simulink subsystem "PvtSubSys_VIE"  (R2020b)
settings: Solver=VariableStepAuto  StartTime=0.0  StopTime=10.0  RelTol=1e-3
undefined symbols (not defined in the file): P_Global_CharSpd_ms, P_Global_FrontAxleToCenter_m, P_Global_RearAxleToCenter_m, P_Global_SideSlipAnglefactor, P_Global_SteeringAngleRatio, P_Global_WheelBase_m, P_Global_WheelTrack_m
libraries: simulink x16
(part 1 of 2)
settings Model: Creator=GW00184765  LastModifiedBy=GW00201118

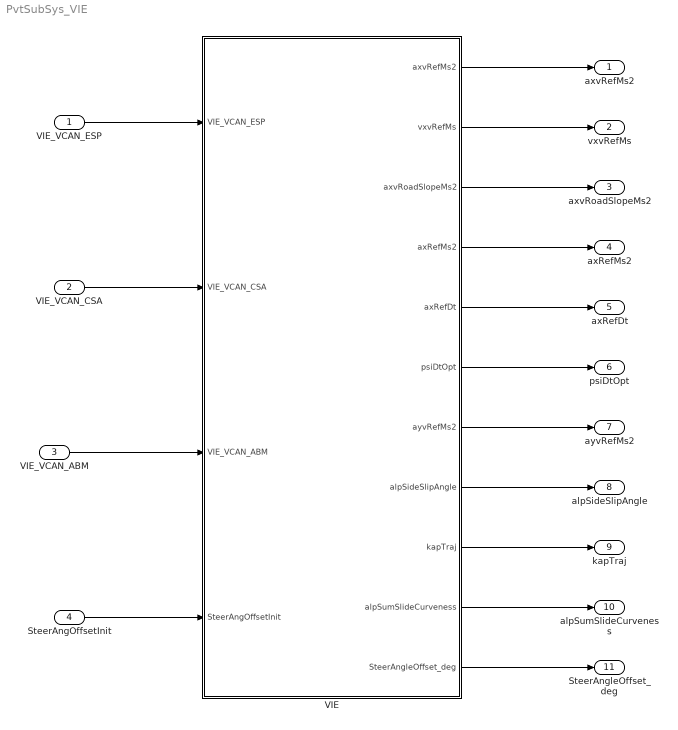
== system PvtSubSys_VIE ==
  VIE_VCAN_ESP : Inport  OutDataTypeStr=Bus: VCAN_ESP_MSG_BUS  PortDimensions=1  BusOutputAsStruct=on
  VIE_VCAN_CSA : Inport  Port=2  OutDataTypeStr=Bus: VCAN_CSA_MSG_BUS  PortDimensions=1  BusOutputAsStruct=on
  VIE_VCAN_ABM : Inport  Port=3  OutDataTypeStr=Bus: VCAN_ABM_MSG_BUS  PortDimensions=1  BusOutputAsStruct=on
  SteerAngOffsetInit : Inport  Port=4
  VIE : Subsystem
  axvRefMs2 : Outport  OutDataTypeStr=single  PortDimensions=1  BusOutputAsStruct=on
  vxvRefMs : Outport  Port=2  OutDataTypeStr=single  PortDimensions=1  BusOutputAsStruct=on
  axvRoadSlopeMs2 : Outport  Port=3  OutDataTypeStr=single  PortDimensions=1  BusOutputAsStruct=on
  axRefMs2 : Outport  Port=4  OutDataTypeStr=single  PortDimensions=1  BusOutputAsStruct=on
  axRefDt : Outport  Port=5  OutDataTypeStr=single  PortDimensions=1  BusOutputAsStruct=on
  psiDtOpt : Outport  Port=6  OutDataTypeStr=single  PortDimensions=1  BusOutputAsStruct=on
  ayvRefMs2 : Outport  Port=7  OutDataTypeStr=single  PortDimensions=1  BusOutputAsStruct=on
  alpSideSlipAngle : Outport  Port=8  OutDataTypeStr=single  PortDimensions=1  BusOutputAsStruct=on
  kapTraj : Outport  Port=9  OutDataTypeStr=single  PortDimensions=1  BusOutputAsStruct=on
  alpSumSlideCurveness : Outport  Port=10  OutDataTypeStr=single  PortDimensions=1  BusOutputAsStruct=on
  SteerAngleOffset_deg : Outport  Port=11  OutDataTypeStr=single  PortDimensions=1  BusOutputAsStruct=on
  wires:
  VIE_VCAN_ABM/1 -> VIE/3(VIE_VCAN_ABM)
  VIE_VCAN_CSA/1 -> VIE/2(VIE_VCAN_CSA)
  VIE_VCAN_ESP/1 -> VIE/1(VIE_VCAN_ESP)
  VIE/9(kapTraj) -> kapTraj/1
  VIE/11(SteerAngleOffset_deg) -> SteerAngleOffset_deg/1
  VIE/8(alpSideSlipAngle) -> alpSideSlipAngle/1
  VIE/7(ayvRefMs2) -> ayvRefMs2/1
  VIE/2(vxvRefMs) -> vxvRefMs/1
  VIE/5(axRefDt) -> axRefDt/1
  VIE/4(axRefMs2) -> axRefMs2/1
  VIE/10(alpSumSlideCurveness) -> alpSumSlideCurveness/1
  VIE/3(axvRoadSlopeMs2) -> axvRoadSlopeMs2/1
  VIE/1(axvRefMs2) -> axvRefMs2/1
  VIE/6(psiDtOpt) -> psiDtOpt/1
  SteerAngOffsetInit/1 -> VIE/4(SteerAngOffsetInit)

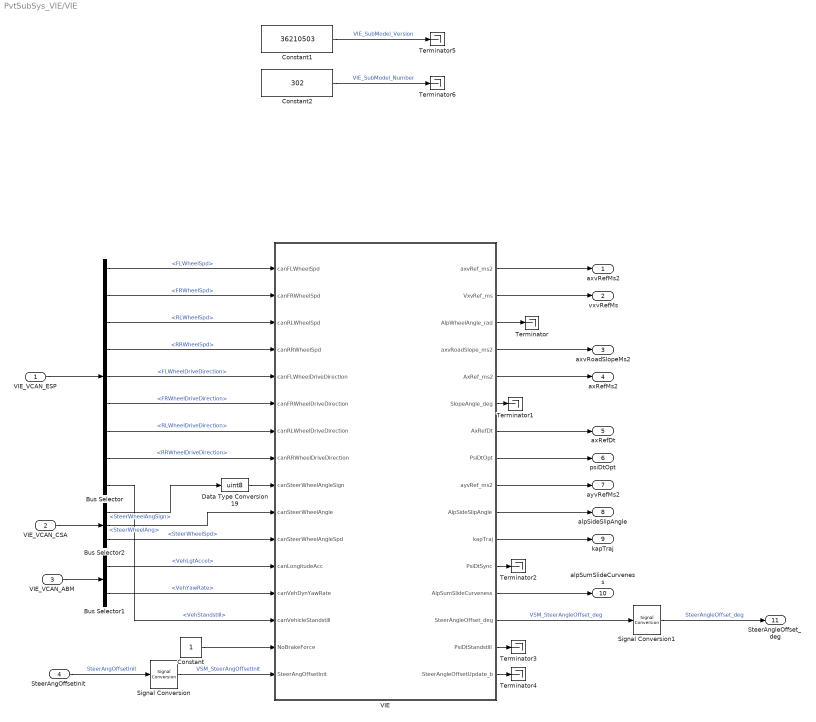
== system PvtSubSys_VIE/VIE ==
  VIE_VCAN_ESP : Inport  OutDataTypeStr=Bus: VCAN_ESP_MSG_BUS  PortDimensions=1  BusOutputAsStruct=on
  VIE_VCAN_CSA : Inport  Port=2  OutDataTypeStr=Bus: VCAN_CSA_MSG_BUS  PortDimensions=1  BusOutputAsStruct=on
  VIE_VCAN_ABM : Inport  Port=3  OutDataTypeStr=Bus: VCAN_ABM_MSG_BUS  PortDimensions=1  BusOutputAsStruct=on
  SteerAngOffsetInit : Inport  Port=4
  Bus Selector : BusSelector  OutputSignals=FLWheelSpd,FRWheelSpd,RLWheelSpd,RRWheelSpd,FLWheelDriveDirection,FRWheelDriveDirection,RLWheelDriveDirection,RRWheelDriveDirection,VehStandstill
  Bus Selector1 : BusSelector  OutputSignals=VehLgtAccel,VehYawRate
  Bus Selector2 : BusSelector  OutputSignals=SteerWheelAngSign,SteerWheelAng,SteerWheelSpd
  Constant : Constant  OutDataTypeStr=single
  Constant1 : Constant  Value=36210503  OutDataTypeStr=uint32
  Constant2 : Constant  Value=302  OutDataTypeStr=uint32
  Data Type Conversion19 : DataTypeConversion  OutDataTypeStr=uint8
  Signal Conversion : SignalConversion  OverrideOpt=off
  Signal Conversion1 : SignalConversion  OverrideOpt=off
  Terminator{,1..6} (7 alike) : Terminator
  VIE : Subsystem
  axvRefMs2 : Outport  OutDataTypeStr=single  PortDimensions=1  BusOutputAsStruct=on
  vxvRefMs : Outport  Port=2  OutDataTypeStr=single  PortDimensions=1  BusOutputAsStruct=on
  axvRoadSlopeMs2 : Outport  Port=3  OutDataTypeStr=single  PortDimensions=1  BusOutputAsStruct=on
  axRefMs2 : Outport  Port=4  OutDataTypeStr=single  PortDimensions=1  BusOutputAsStruct=on
  axRefDt : Outport  Port=5  OutDataTypeStr=single  PortDimensions=1  BusOutputAsStruct=on
  psiDtOpt : Outport  Port=6  OutDataTypeStr=single  PortDimensions=1  BusOutputAsStruct=on
  ayvRefMs2 : Outport  Port=7  OutDataTypeStr=single  PortDimensions=1  BusOutputAsStruct=on
  alpSideSlipAngle : Outport  Port=8  OutDataTypeStr=single  PortDimensions=1  BusOutputAsStruct=on
  kapTraj : Outport  Port=9  OutDataTypeStr=single  PortDimensions=1  BusOutputAsStruct=on
  alpSumSlideCurveness : Outport  Port=10  OutDataTypeStr=single  PortDimensions=1  BusOutputAsStruct=on
  SteerAngleOffset_deg : Outport  Port=11  OutDataTypeStr=single  PortDimensions=1  BusOutputAsStruct=on
  wires:
  VIE/14(SteerAngleOffset_deg) -> Signal Conversion1/1  "VSM_SteerAngleOffset_deg"
  Signal Conversion/1 -> VIE/16(SteerAngOffsetInit)  "VSM_SteerAngOffsetInit"
  Constant1/1 -> Terminator5/1  "VIE_SubModel_Version"
  Constant2/1 -> Terminator6/1  "VIE_SubModel_Number"
  SteerAngOffsetInit/1 -> Signal Conversion/1  "SteerAngOffsetInit"
  VIE/15(PsiDtStandstill) -> Terminator3/1
  VIE/3(AlpWheelAngle_rad) -> Terminator/1
  Signal Conversion1/1 -> SteerAngleOffset_deg/1  "SteerAngleOffset_deg"
  VIE/13(AlpSumSlideCurveness) -> alpSumSlideCurveness/1
  Data Type Conversion19/1 -> VIE/9(canSteerWheelAngleSign)
  VIE/4(axvRoadSlope_ms2) -> axvRoadSlopeMs2/1
  VIE/6(SlopeAngle_deg) -> Terminator1/1
  VIE/10(AlpSideSlipAngle) -> alpSideSlipAngle/1
  VIE/5(AxRef_ms2) -> axRefMs2/1
  VIE/11(kapTraj) -> kapTraj/1
  VIE/7(AxRefDt) -> axRefDt/1
  VIE/8(PsiDtOpt) -> psiDtOpt/1
  Bus Selector/7 -> VIE/7(canRLWheelDriveDirection)  "<RLWheelDriveDirection>"
  Bus Selector/6 -> VIE/6(canFRWheelDriveDirection)  "<FRWheelDriveDirection>"
  VIE_VCAN_ABM/1 -> Bus Selector1/1
  Constant/1 -> VIE/15(NoBrakeForce)
  Bus Selector/8 -> VIE/8(canRRWheelDriveDirection)  "<RRWheelDriveDirection>"
  VIE/12(PsiDtSync) -> Terminator2/1
  Bus Selector1/2 -> VIE/13(canVehDynYawRate)  "<VehYawRate>"
  Bus Selector2/3 -> VIE/11(canSteerWheelAngleSpd)  "<SteerWheelSpd>"
  Bus Selector2/1 -> Data Type Conversion19/1  "<SteerWheelAngSign>"
  VIE/9(ayvRef_ms2) -> ayvRefMs2/1
  Bus Selector/9 -> VIE/14(canVehicleStandstill)  "<VehStandstill>"
  Bus Selector2/2 -> VIE/10(canSteerWheelAngle)  "<SteerWheelAng>"
  Bus Selector/5 -> VIE/5(canFLWheelDriveDirection)  "<FLWheelDriveDirection>"
  VIE_VCAN_CSA/1 -> Bus Selector2/1
  Bus Selector/3 -> VIE/3(canRLWheelSpd)  "<RLWheelSpd>"
  VIE/2(VxvRef_ms) -> vxvRefMs/1
  Bus Selector1/1 -> VIE/12(canLongitudeAcc)  "<VehLgtAccel>"
  Bus Selector/1 -> VIE/1(canFLWheelSpd)  "<FLWheelSpd>"
  VIE/16(SteerAngleOffsetUpdate_b) -> Terminator4/1
  VIE/1(axvRef_ms2) -> axvRefMs2/1
  Bus Selector/2 -> VIE/2(canFRWheelSpd)  "<FRWheelSpd>"
  VIE_VCAN_ESP/1 -> Bus Selector/1
  Bus Selector/4 -> VIE/4(canRRWheelSpd)  "<RRWheelSpd>"

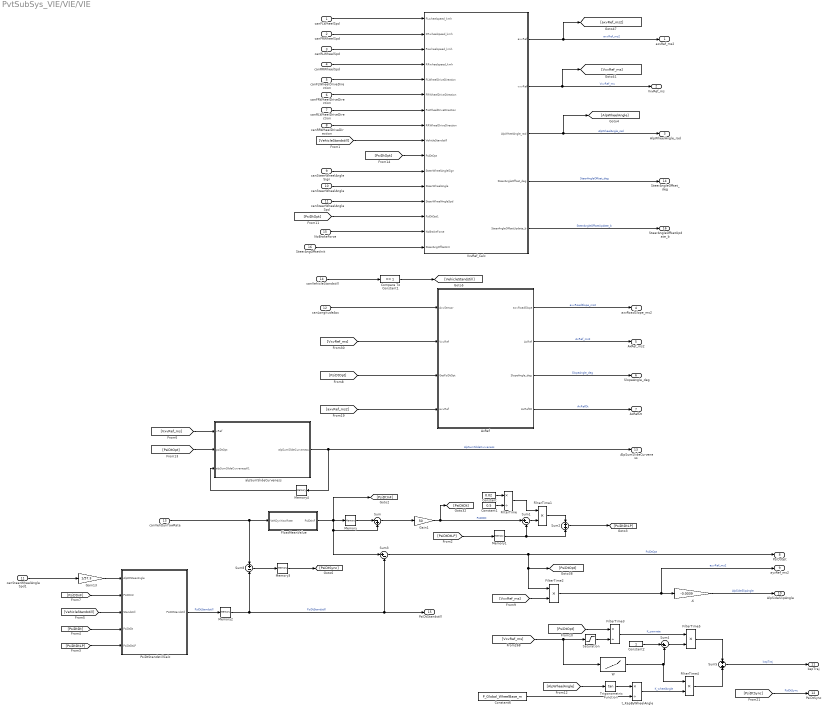
== system PvtSubSys_VIE/VIE/VIE ==
  canFLWheelSpd : Inport
  canFRWheelSpd : Inport  Port=2
  canRLWheelSpd : Inport  Port=3
  canRRWheelSpd : Inport  Port=4
  canFLWheelDriveDirection : Inport  Port=5
  canFRWheelDriveDirection : Inport  Port=6
  canRLWheelDriveDirection : Inport  Port=7
  canRRWheelDriveDirection : Inport  Port=8
  canSteerWheelAngleSign : Inport  Port=9
  canSteerWheelAngle : Inport  Port=10
  canSteerWheelAngleSpd : Inport  Port=11
  canLongitudeAcc : Inport  Port=12
  canVehDynYawRate : Inport  Port=13
  canVehicleStandstill : Inport  Port=14
  NoBrakeForce : Inport  Port=15
  SteerAngOffsetInit : Inport  Port=16
  -K : Gain  Gain=-0.0039
  AxRef : Subsystem
  Compare To Constant1 : simulink/Logic and Bit Operations/Compare To Constant  relop===  const=1  OutDataTypeStr=boolean
  Constant : Constant  Value=0.02  OutDataTypeStr=single
  Constant1 : Constant  Value=0.5  OutDataTypeStr=single
  Constant2 : Constant  OutDataTypeStr=single
  Constant6 : Constant  Value=P_Global_WheelBase_m
  FilterTime : Product  Inputs=*/  RndMeth=Zero
  FilterTime{1..2,4..5} (4 alike) : Product  RndMeth=Zero
  FilterTime3 : Product  Inputs=*/  RndMeth=Zero
  FloatMeanValue : Subsystem
  Gain1 : Gain  Gain=50
  Gain13 : Gain  Gain=1/57.3
  Memory{,1..4} (5 alike) : Memory  InheritSampleTime=on
  PsiDtStandstillCalc : Subsystem  TreatAsAtomicUnit=on
  Saturation : Saturate  UpperLimit=200  LowerLimit=0.5
  Sum : Sum  Inputs=|-+
  Sum1 : Sum  Inputs=|+-
  Sum2 : Sum
  Sum3 : Sum  Inputs=|+-
  Sum4 : Sum  Inputs=|+-
  Sum5 : Sum
  Sum8 : Sum  Inputs=+-
  Trigonometric Function : Trigonometry  Operator=tan
  VxvRef_Calc : Subsystem
  W : Lookup_n-D  NumberOfTableDimensions=1  BreakpointsForDimension1=[0,1,1.5,3]  Table=[1,1,0,0]  RndMeth=Simplest  InputSameDT=on
  alpSumSlideCurveness : MATLAB Function  TreatAsAtomicUnit=on
  canSteerWheelAngleSpd1 : InportShadow  Port=11
  t_KapByWheelAngle : Product  Inputs=*/  RndMeth=Zero
  axvRef_ms2 : Outport
  VxvRef_ms : Outport  Port=2
  AlpWheelAngle_rad : Outport  Port=3
  axvRoadSlope_ms2 : Outport  Port=4
  AxRef_ms2 : Outport  Port=5
  SlopeAngle_deg : Outport  Port=6
  AxRefDt : Outport  Port=7
  PsiDtOpt : Outport  Port=8
  ayvRef_ms2 : Outport  Port=9
  AlpSideSlipAngle : Outport  Port=10
  kapTraj : Outport  Port=11
  PsiDtSync : Outport  Port=12
  AlpSumSlideCurveness : Outport  Port=13
  SteerAngleOffset_deg : Outport  Port=14
  PsiDtStandstill : Outport  Port=15
  SteerAngleOffsetUpdate_b : Outport  Port=16
  wires:
  [PsiDtOpt] -> VxvRef_Calc/10(PsiDtOpt)
  SteerAngOffsetInit/1 -> VxvRef_Calc/16(SteerAngOffsetInit)
  Sum/1 -> Gain1/1
  Memory/1 -> Sum/1
  FloatMeanValue/1(PsiDtInF) -> [PsiDtInF], Memory/1, Sum3/1, Sum/2
  Memory4/1 -> alpSumSlideCurveness/3(alpSumSlideCurvenessK1)
  NoBrakeForce/1 -> VxvRef_Calc/15(NoBrakeForce)
  VxvRef_Calc/5(SteerAngleOffsetUpdate_b) -> SteerAngleOffsetUpdate_b/1  "SteerAngleOffsetUpdate_b"
  canSteerWheelAngleSpd/1 -> VxvRef_Calc/13(SteerWheelAngleSpd)
  VxvRef_Calc/4(SteerAngleOffset_deg) -> SteerAngleOffset_deg/1  "SteerAngleOffset_deg"
  [PsiDtOpt] -> alpSumSlideCurveness/2(psiDtOpt)
  [VxvRef_ms] -> alpSumSlideCurveness/1(vRef)
  alpSumSlideCurveness/1(alpSumSlideCurveness) -> Memory4/1, AlpSumSlideCurveness/1  "AlpSumSlideCurveness"
  Compare To Constant1/1 -> [VehicleStandstill]
  Memory2/1 -> Sum8/2, Sum3/2, PsiDtStandstill/1  "PsiDtStandstill"
  canFLWheelDriveDirection/1 -> VxvRef_Calc/5(FLWheelDriveDirection)
  canRLWheelDriveDirection/1 -> VxvRef_Calc/7(RLWheelDriveDirection)
  Memory3/1 -> [PsiDtSync]
  [PsiDtDtLP] -> PsiDtStandstillCalc/5(PsiDtDtLP)
  AxRef/4(AxRefDt) -> AxRefDt/1  "AxRefDt"
  Gain1/1 -> Sum1/1, [PsiDtDt]  "PsiDtDt"
  [PsiDtDt] -> PsiDtStandstillCalc/4(PsiDtDt)
  canLongitudeAcc/1 -> AxRef/1(AxvSensor)
  FilterTime/1 -> FilterTime1/1
  Memory1/1 -> Sum1/2, Sum2/2
  Sum8/1 -> Memory3/1
  [VxvRef_ms] -> FilterTime2/2
  FilterTime5/1 -> Sum5/1
  AxRef/3(SlopeAngle_deg) -> SlopeAngle_deg/1  "SlopeAngle_deg"
  VxvRef_Calc/2(vxvRef) -> VxvRef_ms/1, [VxvRef_ms]  "VxvRef_ms"
  [PsiDtOpt] -> VxvRef_Calc/14(PsiDtOpt1)
  Sum3/1 -> [PsiDtOpt], FilterTime2/1, PsiDtOpt/1  "PsiDtOpt"
  [VehicleStandstill] -> PsiDtStandstillCalc/3(Standstill)
  [PsiDtSync] -> PsiDtSync/1  "PsiDtSync"
  Sum1/1 -> FilterTime1/2
  [PsiDtInF] -> PsiDtStandstillCalc/2(PsiDtInF)
  canSteerWheelAngle/1 -> VxvRef_Calc/12(SteerWheelAngle)
  [VxvRef_ms] -> AxRef/2(VxvRef)
  AxRef/2(AxRef) -> AxRef_ms2/1  "AxRef_ms2"
  canRRWheelSpd/1 -> VxvRef_Calc/4(RRwheelspeed_kmh)
  canRRWheelDriveDirection/1 -> VxvRef_Calc/8(RRWheelDriveDirection)
  VxvRef_Calc/3(AlpWheelAngle_rad) -> AlpWheelAngle_rad/1, [AlpWheelAngle]  "AlpWheelAngle_rad"
  canSteerWheelAngleSign/1 -> VxvRef_Calc/11(SteerWheelAngleSign)
  Constant/1 -> FilterTime/1
  FilterTime1/1 -> Sum2/1
  PsiDtStandstillCalc/1(PsiDtStandstill) -> Memory2/1  "PsiDtStandstill"
  [PsiDtOpt] -> AxRef/3(GetPsiDtOpt)
  canFRWheelSpd/1 -> VxvRef_Calc/2(FRwheelspeed_kmh)
  FilterTime2/1 -> ayvRef_ms2/1, -K/1  "ayvRef_ms2"
  [AlpWheelAngle] -> Trigonometric Function/1
  canRLWheelSpd/1 -> VxvRef_Calc/3(RLwheelspeed_kmh)
  Trigonometric Function/1 -> t_KapByWheelAngle/1
  Constant2/1 -> Sum4/1
  W/1 -> FilterTime4/1, Sum4/2
  canFRWheelDriveDirection/1 -> VxvRef_Calc/6(FRWheelDriveDirection)
  FilterTime4/1 -> Sum5/2
  canSteerWheelAngleSpd1/1 -> Gain13/1
  canVehDynYawRate/1 -> FloatMeanValue/1(VehDynYawRate), Sum8/1
  canFLWheelSpd/1 -> VxvRef_Calc/1(FLwheelspeed_kmh)
  t_KapByWheelAngle/1 -> FilterTime4/2  "K_wheelAngle"
  [PsiDtOpt] -> FilterTime3/1
  VxvRef_Calc/1(axvRef) -> axvRef_ms2/1, [axvRef_ms2]  "axvRef_ms2"
  Saturation/1 -> FilterTime3/2
  Constant1/1 -> FilterTime/2
  canVehicleStandstill/1 -> Compare To Constant1/1
  Gain13/1 -> PsiDtStandstillCalc/1(AlpDtSteerAngle)
  Constant6/1 -> t_KapByWheelAngle/2
  [axvRef_ms2] -> AxRef/4(axvRef)
  AxRef/1(axvRoadSlope) -> axvRoadSlope_ms2/1  "axvRoadSlope_ms2"
  Sum4/1 -> FilterTime5/2
  Sum2/1 -> [PsiDtDtLP]
  [PsiDtDtLP] -> Memory1/1
  [VxvRef_ms] -> W/1, Saturation/1
  FilterTime3/1 -> FilterTime5/1  "K_yawrate"
  Sum5/1 -> kapTraj/1  "kapTraj"
  [VehicleStandstill] -> VxvRef_Calc/9(VehicleStandstill)
  -K/1 -> AlpSideSlipAngle/1  "AlpSideSlipAngle"

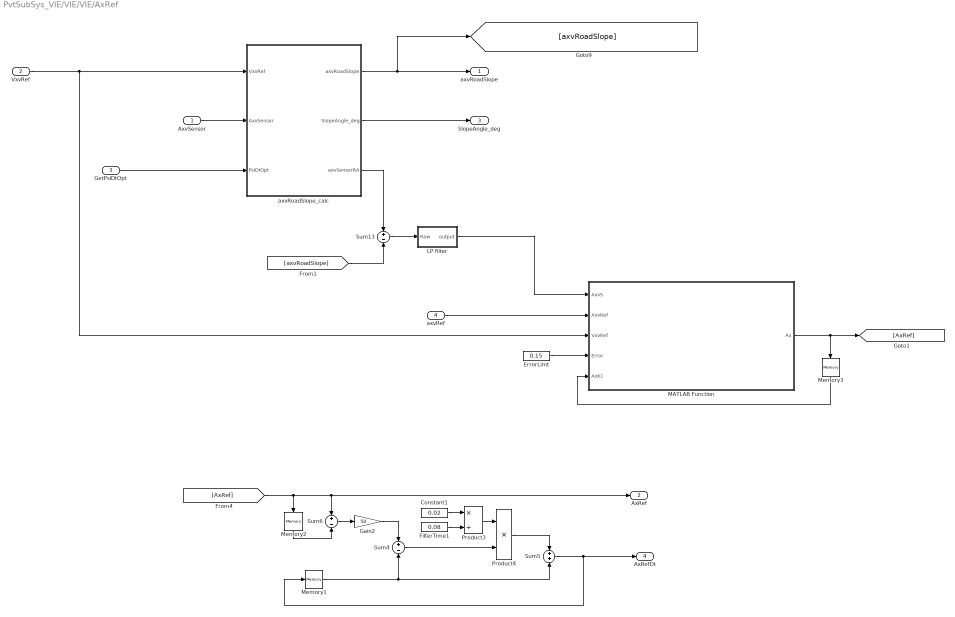
== system PvtSubSys_VIE/VIE/VIE/AxRef ==
  AxvSensor : Inport
  VxvRef : Inport  Port=2
  GetPsiDtOpt : Inport  Port=3
  axvRef : Inport  Port=4
  Constant1 : Constant  Value=0.02  OutDataTypeStr=single
  ErrorLimt : Constant  Value=0.15  OutDataTypeStr=single
  FilterTime1 : Constant  Value=0.08  OutDataTypeStr=single
  Gain2 : Gain  Gain=50
  LP filter : Subsystem
  MATLAB Function : MATLAB Function  TreatAsAtomicUnit=on
  Memory1 : Memory  InheritSampleTime=on
  Memory2 : Memory  InheritSampleTime=on
  Memory3 : Memory  InheritSampleTime=on
  Product3 : Product  Inputs=*/  RndMeth=Zero
  Product4 : Product  RndMeth=Zero
  Sum13 : Sum  Inputs=+-
  Sum4 : Sum  Inputs=+-
  Sum5 : Sum
  Sum6 : Sum  Inputs=+-
  axvRoadSlope_calc : Subsystem
  axvRoadSlope : Outport
  AxRef : Outport  Port=2
  SlopeAngle_deg : Outport  Port=3
  AxRefDt : Outport  Port=4
  wires:
  ErrorLimt/1 -> MATLAB Function/4(Error)
  Memory3/1 -> MATLAB Function/5(AxK1)
  MATLAB Function/1(Ax) -> [AxRef], Memory3/1
  [AxRef] -> Memory2/1, AxRef/1, Sum6/1
  LP filter/1(output) -> MATLAB Function/1(AxvS)
  Gain2/1 -> Sum4/1
  Sum6/1 -> Gain2/1
  Memory2/1 -> Sum6/2
  Product4/1 -> Sum5/1
  Product3/1 -> Product4/1
  Sum4/1 -> Product4/2
  FilterTime1/1 -> Product3/2
  Constant1/1 -> Product3/1
  Memory1/1 -> Sum4/2, Sum5/2
  Sum5/1 -> Memory1/1, AxRefDt/1
  axvRoadSlope_calc/1(axvRoadSlope) -> [axvRoadSlope], axvRoadSlope/1
  axvRef/1 -> MATLAB Function/2(AxvRef)
  axvRoadSlope_calc/2(SlopeAngle_deg) -> SlopeAngle_deg/1
  axvRoadSlope_calc/3(axvSensorRA) -> Sum13/1
  [axvRoadSlope] -> Sum13/2
  VxvRef/1 -> axvRoadSlope_calc/1(VxvRef), MATLAB Function/3(VxvRef)
  Sum13/1 -> LP filter/1(Raw)
  GetPsiDtOpt/1 -> axvRoadSlope_calc/3(PsiDtOpt)
  AxvSensor/1 -> axvRoadSlope_calc/2(AxvSensor)

== system PvtSubSys_VIE/VIE/VIE/FloatMeanValue ==
  VehDynYawRate : Inport
  Gain : Gain  Gain=0.2
  Sum of Elements : Sum  Inputs=+
  Tapped Delay : simulink/Discrete/Tapped Delay  vinit=0.0  samptime=-1  NumDelays=4  DelayOrder=Newest  includeCurrent=on
  PsiDtInF : Outport
  wires:
  Sum of Elements/1 -> Gain/1
  VehDynYawRate/1 -> Tapped Delay/1
  Gain/1 -> PsiDtInF/1  "PsiDtInF"
  Tapped Delay/1 -> Sum of Elements/1

== system PvtSubSys_VIE/VIE/VIE/PsiDtStandstillCalc ==
  AlpDtSteerAngle : Inport
  PsiDtInF : Inport  Port=2
  Standstill : Inport  Port=3
  PsiDtDt : Inport  Port=4
  PsiDtDtLP : Inport  Port=5
  MATLAB Function : MATLAB Function  TreatAsAtomicUnit=on
  Memory2 : Memory  InheritSampleTime=on
  Memory3 : Memory  InheritSampleTime=on
  PsiDtStandstill : Outport
  wires:
  Memory2/1 -> MATLAB Function/6(PsiDtLPK1)
  MATLAB Function/1(PsiDtLP) -> Memory2/1
  AlpDtSteerAngle/1 -> MATLAB Function/1(AlpDtSteerAngle)
  MATLAB Function/2(PsiDtStandstill) -> Memory3/1, PsiDtStandstill/1
  PsiDtInF/1 -> MATLAB Function/2(PsiDtInF)
  Standstill/1 -> MATLAB Function/3(Standstill)
  PsiDtDt/1 -> MATLAB Function/4(PsiDtDt)
  PsiDtDtLP/1 -> MATLAB Function/5(PsiDtDtLP)
  Memory3/1 -> MATLAB Function/7(PsiDtStandstillK1)

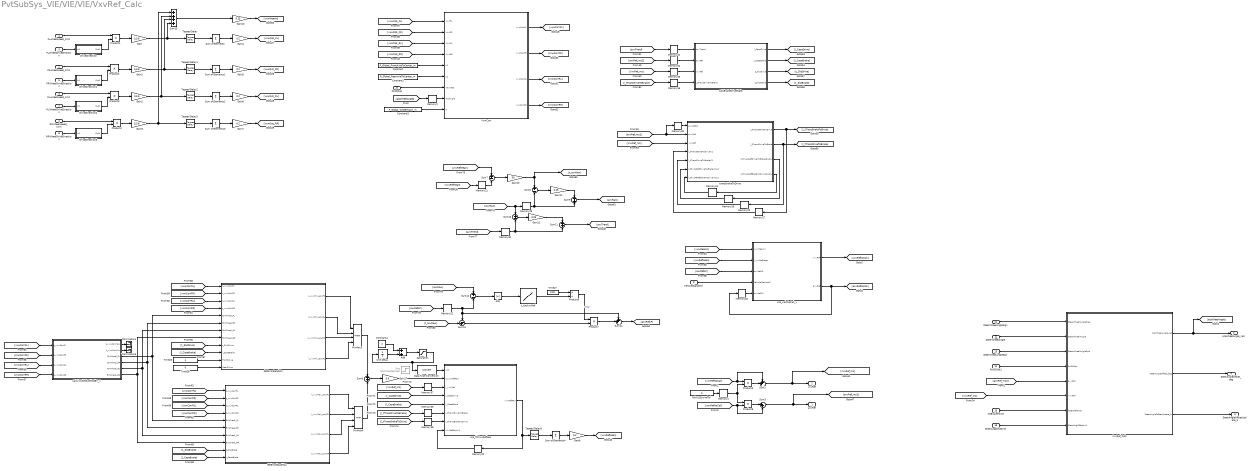
== system PvtSubSys_VIE/VIE/VIE/VxvRef_Calc ==
  FLwheelspeed_kmh : Inport
  FRwheelspeed_kmh : Inport  Port=2
  RLwheelspeed_kmh : Inport  Port=3
  RRwheelspeed_kmh : Inport  Port=4
  FLWheelDriveDirection : Inport  Port=5
  FRWheelDriveDirection : Inport  Port=6
  RLWheelDriveDirection : Inport  Port=7
  RRWheelDriveDirection : Inport  Port=8
  VehicleStandstill : Inport  Port=9
  PsiDtOpt : Inport  Port=10
  SteerWheelAngleSign : Inport  Port=11
  SteerWheelAngle : Inport  Port=12
  SteerWheelAngleSpd : Inport  Port=13
  PsiDtOpt1 : Inport  Port=14
  NoBrakeForce : Inport  Port=15
  SteerAngOffsetInit : Inport  Port=16
  Abs : Abs
  Add : Sum
  Constant : Constant  Value=P_Global_FrontAxleToCenter_m  OutDataTypeStr=single
  Constant1 : Constant
  Constant2 : Constant  Value=P_Global_RearAxleToCenter_m  OutDataTypeStr=single
  Constant3 : Constant  Value=P_Global_WheelTrack_m  OutDataTypeStr=single
  Data Type Conversion : DataTypeConversion
  DriveDirection : Subsystem
  DriveDirection1 : Subsystem
  DriveDirection2 : Subsystem
  DriveDirection3 : Subsystem
  Fak0125sVrefTol : Constant  Value=0  OutDataTypeStr=single
  Gain{,1..3} (4 alike) : Gain  Gain=1/3.6
  Gain10 : Gain  Gain=50
  Gain11 : Gain  Gain=0.25
  Gain12 : Gain  Gain=0.05
  Gain13 : Gain  Gain=0.25
  Gain17 : Gain  Gain=0.5
  Gain{4..8} (5 alike) : Gain  Gain=0.2
  Memory{1..2,21..31,33..39} (20 alike) : Memory  InheritSampleTime=on
  MinMax3 : MinMax  Function=max  Inputs=4
  MinMax4 : MinMax  Inputs=4
  Product{1..5,7..8} (7 alike) : Product  RndMeth=Zero
  Product6 : Product  Inputs=*/  RndMeth=Zero
  Saturation : Saturate  UpperLimit=2  LowerLimit=0
  Step : Step  Commented=on  Time=0.1  Before=1  After=0
  Sum of Elements{,1..4} (5 alike) : Sum  Inputs=+
  Sum{7..8,10,12} (4 alike) : Sum  Inputs=+-
  Sum11 : Sum
  Sum13 : Sum  Inputs=-+|
  Sum14 : Sum  Inputs=++|
  Sum15 : Sum  Inputs=++++
  Sum2 : Sum  Inputs=++|
  Sum3 : Sum  Inputs=|++
  Sum6 : Sum
  Sum9 : Sum
  Tapped Delay{,1..3,8} (5 alike) : simulink/Discrete/Tapped Delay  vinit=0.0  samptime=-1  NumDelays=4  DelayOrder=Newest  includeCurrent=on
  Terminator4 : Terminator
  Terminator5 : Terminator
  Time25 : Constant  OutDataTypeStr=uint8
  Time26 : Constant  Value=0  OutDataTypeStr=uint8
  Time27 : Constant  Value=0.02  OutDataTypeStr=single
  Unit Delay : UnitDelay  SampleTime=-1  HasFrameUpgradeWarning=on
  VxvRef_Calc : Subsystem
  VxwCorr : MATLAB Function  TreatAsAtomicUnit=on
  calcBrakeDriveState : MATLAB Function  TreatAsAtomicUnit=on
  calcVxwDiffAndModErr_v : MATLAB Function  TreatAsAtomicUnit=on
  detErrorBandMax : MATLAB Function  TreatAsAtomicUnit=on
  detErrorBandMin : MATLAB Function  TreatAsAtomicUnit=on
  t_tauAxvRef : Lookup_n-D  NumberOfTableDimensions=1  BreakpointsForDimension1=[0,1,2]  Table=[0.2,0.1,0.1]  RndMeth=Simplest  InputSameDT=on
  transBrakeToDrive : MATLAB Function  TreatAsAtomicUnit=on
  vsp_calcNoCali_v : MATLAB Function  TreatAsAtomicUnit=on
  vsp_filtVxvRefRaw : MATLAB Function  TreatAsAtomicUnit=on
  axvRef : Outport
  vxvRef : Outport  Port=2
  AlpWheelAngle_rad : Outport  Port=3
  SteerAngleOffset_deg : Outport  Port=4
  SteerAngleOffsetUpdate_b : Outport  Port=5
  wires:
  SteerAngOffsetInit/1 -> VxvRef_Calc/8(SteerAngOffsetInit)
  NoBrakeForce/1 -> VxvRef_Calc/7(NoBrakeForce)
  VxvRef_Calc/3(SteerAngleOffsetUpdate_b) -> SteerAngleOffsetUpdate_b/1
  VxvRef_Calc/1(AlpWheelAngle_rad) -> AlpWheelAngle_rad/1, [alpWheelAngle]
  VxvRef_Calc/2(SteerAngleOffset_deg) -> SteerAngleOffset_deg/1
  [VxvRef_ms] -> VxvRef_Calc/6(vxvRef)
  [axvRef_ms2] -> VxvRef_Calc/5(axvRef)
  PsiDtOpt1/1 -> VxvRef_Calc/4(PsiDtOpt)
  SteerWheelAngleSpd/1 -> VxvRef_Calc/3(SteerWheelAngleSpd)
  SteerWheelAngleSign/1 -> VxvRef_Calc/1(SteerWheelAngleSign)
  SteerWheelAngle/1 -> VxvRef_Calc/2(SteerWheelAngle)
  Saturation/1 -> Unit Delay/1, Data Type Conversion/1
  Constant1/1 -> Add/1
  Unit Delay/1 -> Add/2
  Data Type Conversion/1 -> vsp_filtVxvRefRaw/1(Init)
  Sum of Elements3/1 -> Gain7/1
  Sum of Elements2/1 -> Gain6/1
  Sum of Elements1/1 -> Gain5/1
  Sum of Elements/1 -> Gain4/1
  Gain4/1 -> [vxwOpt_FL]
  [vxwOpt_RL] -> VxwCorr/3(VxwRL)
  detErrorBandMin/1(l_vxwMin_aswFR) -> MinMax3/1
  Add/1 -> Saturation/1
  Memory2/1 -> VxwCorr/8(alpAngle)
  [alpWheelAngle] -> Memory2/1
  Memory1/1 -> Product8/1, Product5/2
  Sum3/1 -> axvRef/1, [axvRef_ms2]
  Sum2/1 -> vxvRef/1, [VxvRef_ms]
  Product8/1 -> Sum3/1
  Product5/1 -> Sum2/2
  [axvRefNoCali] -> Sum3/2, Product8/2
  [vxvRefNoCali] -> Sum2/1, Product5/1
  Fak0125sVrefTol/1 -> Memory1/1
  vsp_calcNoCali_v/1(vxvRef) -> [vxvRefNoCali]
  vsp_calcNoCali_v/2(axvRef) -> Memory33/1, [axvRefNoCali]
  DriveDirection3/1(Out1) -> Product4/2
  Product4/1 -> Gain3/1
  DriveDirection2/1(Out1) -> Product3/2
  Product3/1 -> Gain2/1
  Product2/1 -> Gain1/1
  DriveDirection1/1(Out1) -> Product2/2
  Product1/1 -> Gain/1
  DriveDirection/1(Out1) -> Product1/2
  RRWheelDriveDirection/1 -> DriveDirection3/1(In1)
  RLWheelDriveDirection/1 -> DriveDirection2/1(In1)
  FRWheelDriveDirection/1 -> DriveDirection1/1(In1)
  FLWheelDriveDirection/1 -> DriveDirection/1(In1)
  Sum of Elements4/1 -> Gain8/1
  Memory38/1 -> vsp_filtVxvRefRaw/7(l_tTransBrakeToDrive)
  Memory39/1 -> vsp_filtVxvRefRaw/6(l_tTransDriveToBrake)
  Memory37/1 -> vsp_filtVxvRefRaw/3(l_vxvRef)
  Memory36/1 -> calcBrakeDriveState/4(l_tTransDriveToBrake)
  Memory35/1 -> calcBrakeDriveState/3(vxvRef)
  Memory34/1 -> calcBrakeDriveState/2(axvRef)
  Memory31/1 -> calcBrakeDriveState/1(axvTrend)
  Memory22/1 -> Sum12/2, Sum14/1, Sum13/1
  [axvRefLP] -> Memory22/1
  Memory21/1 -> Sum7/2
  vsp_filtVxvRefRaw/1(vxvRefRaw) -> Tapped Delay8/1, Memory23/1
  calcVxwDiffAndModErr_v/2(t_vxwCorrMin) -> Terminator5/1
  calcVxwDiffAndModErr_v/1(t_vxwCorrMax) -> Terminator4/1
  [l_tTransDriveToBrake] -> Memory36/1
  Memory33/1 -> vsp_calcNoCali_v/5(axvRefK1)
  VehicleStandstill/1 -> vsp_calcNoCali_v/4(VehicleStandstill)
  [axvRefLP] -> vsp_calcNoCali_v/3(axvRefLP)
  [vxvRefMean] -> vsp_calcNoCali_v/2(l_vxvRefMean)
  [vxwMeanIn] -> vsp_calcNoCali_v/1(vxwMeanIn)
  Sum14/1 -> [axvRefLP]
  Product7/1 -> Sum14/2
  Sum13/1 -> Product7/2
  Product6/1 -> Product7/1  "filter"
  [t_axvRaw] -> Sum13/2
  Time27/1 -> Product6/1
  t_tauAxvRef/1 -> Product6/2
  Abs/1 -> t_tauAxvRef/1
  Sum12/1 -> Abs/1
  [axvRaw] -> Sum12/1
  Sum11/1 -> [axvTrend]
  Gain12/1 -> Sum11/1
  Sum10/1 -> Gain12/1
  Memory30/1 -> Sum10/2, Sum11/2
  [axvTrend] -> Memory30/1
  Memory29/1 -> Sum8/2, Sum9/2
  Sum9/1 -> [axvRaw]
  Gain11/1 -> Sum9/1
  Sum8/1 -> Gain11/1
  [axvRaw] -> Memory29/1, Sum10/1
  Gain10/1 -> [t_axvRaw], Sum8/1
  Sum7/1 -> Gain10/1
  [vxvRefMean] -> Memory21/1
  [vxvRefMean] -> Sum7/1
  [l_tTransDriveToBrake] -> Memory39/1
  [l_tTransBrakeToDrive] -> Memory38/1
  [l_CaseBrake] -> vsp_filtVxvRefRaw/5(l_CaseBrake)
  [l_CaseDrive] -> vsp_filtVxvRefRaw/4(l_CaseDrive)
  [VxvRef_ms] -> Memory37/1
  transBrakeToDrive/1(l_tTransBrakeToDrive) -> [l_tTransBrakeToDrive], Memory27/1
  Time26/1 -> detErrorBandMin/12(RearDrive)
  Time25/1 -> detErrorBandMin/11(FrontDrive)
  [t_SlipBrake] -> detErrorBandMax/9(t_SlipBrake)
  [l_CaseBrake] -> detErrorBandMax/10(l_CaseBrake)
  [l_CaseBrake] -> detErrorBandMin/10(l_CaseBrake)
  [t_SlipDrive] -> detErrorBandMin/9(t_SlipDrive)
  calcBrakeDriveState/4(t_SlipBrake) -> [t_SlipBrake]
  calcBrakeDriveState/3(t_SlipDrive) -> [t_SlipDrive]
  calcBrakeDriveState/2(l_CaseBrake) -> [l_CaseBrake]
  calcBrakeDriveState/1(l_CaseDrive) -> [l_CaseDrive]
  [vxwCorrRR] -> detErrorBandMax/4(t_vxwCorrRR)
  [vxwCorrRL] -> detErrorBandMax/3(t_vxwCorrRL)
  [vxwCorrFR] -> detErrorBandMax/2(t_vxwCorrFR)
  [vxwCorrFL] -> detErrorBandMax/1(t_vxwCorrFL)
  [vxwCorrRR] -> detErrorBandMin/4(t_vxwCorrRR)
  [vxwCorrRL] -> detErrorBandMin/3(t_vxwCorrRL)
  [vxwCorrFR] -> detErrorBandMin/2(t_vxwCorrFR)
  [vxwCorrFL] -> detErrorBandMin/1(t_vxwCorrFL)
  calcVxwDiffAndModErr_v/5(ErrWheel_RL) -> detErrorBandMax/7(ErrWheel_RL), detErrorBandMin/7(ErrWheel_RL)
  calcVxwDiffAndModErr_v/6(ErrWheel_RR) -> detErrorBandMax/8(ErrWheel_RR), detErrorBandMin/8(ErrWheel_RR)
  calcVxwDiffAndModErr_v/4(ErrWheel_FR) -> detErrorBandMax/6(ErrWheel_FR), detErrorBandMin/6(ErrWheel_FR)
  calcVxwDiffAndModErr_v/3(ErrWheel_FL) -> detErrorBandMax/5(ErrWheel_FL), detErrorBandMin/5(ErrWheel_FL)
  [vxwCorrRR] -> calcVxwDiffAndModErr_v/4(t_vxwCorrRR)
  [vxwCorrRL] -> calcVxwDiffAndModErr_v/3(t_vxwCorrRL)
  [vxwCorrFR] -> calcVxwDiffAndModErr_v/2(t_vxwCorrFR)
  [vxwCorrFL] -> calcVxwDiffAndModErr_v/1(t_vxwCorrFL)
  VxwCorr/4(vxwCorrRR) -> [vxwCorrRR]
  VxwCorr/3(vxwCorrRL) -> [vxwCorrRL]
  VxwCorr/2(vxwCorrFR) -> [vxwCorrFR]
  VxwCorr/1(vxwCorrFL) -> [vxwCorrFL]
  Memory28/1 -> transBrakeToDrive/1(axvRefK1)
  [axvRef_ms2] -> Memory28/1, transBrakeToDrive/2(axvRef)
  [VxvRef_ms] -> transBrakeToDrive/3(vxvRef)
  [VxvRef_ms] -> Memory35/1
  [axvRef_ms2] -> Memory34/1
  [axvTrend] -> Memory31/1
  Gain8/1 -> [vxvRefMean]
  Tapped Delay8/1 -> Sum of Elements4/1
  Memory24/1 -> transBrakeToDrive/7(l_tHysARefBrakeToDriveInput)
  Memory26/1 -> transBrakeToDrive/6(l_tHysARefDriveToBrakeInput)
  Memory25/1 -> transBrakeToDrive/5(l_tTransDriveToBrakeK1)
  Memory27/1 -> transBrakeToDrive/4(l_tTransBrakeToDriveK1)
  transBrakeToDrive/2(l_tTransDriveToBrake) -> Memory25/1, [l_tTransDriveToBrake]
  transBrakeToDrive/3(l_tHysARefDriveToBrakeOutput) -> Memory26/1
  transBrakeToDrive/4(l_tHysARefBrakeToDriveOutput) -> Memory24/1
  Memory23/1 -> vsp_filtVxvRefRaw/8(vxvRefRawK1)
  Gain17/1 -> vsp_filtVxvRefRaw/2(t_vxvRefRaw)
  Sum6/1 -> Gain17/1
  MinMax4/1 -> Sum6/2
  MinMax3/1 -> Sum6/1
  detErrorBandMax/4(l_vxwMax_aswRR) -> MinMax4/4
  detErrorBandMax/3(l_vxwMax_aswRL) -> MinMax4/3
  detErrorBandMax/2(l_vxwMax_aswFR) -> MinMax4/2
  detErrorBandMax/1(l_vxwMax_aswFL) -> MinMax4/1
  detErrorBandMin/3(l_vxwMin_aswRR) -> MinMax3/3
  detErrorBandMin/2(l_vxwMin_aswRL) -> MinMax3/2
  detErrorBandMin/4(l_vxwMin_aswFL) -> MinMax3/4
  Constant3/1 -> VxwCorr/9(b)
  PsiDtOpt/1 -> VxwCorr/7(Yawrate)
  Constant2/1 -> VxwCorr/6(L2)
  Constant/1 -> VxwCorr/5(L1)
  [vxwOpt_RR] -> VxwCorr/4(VxwRR)
  [vxwOpt_FR] -> VxwCorr/2(VxwFR)
  [vxwOpt_FL] -> VxwCorr/1(VxwFL)
  Gain/1 -> Sum15/4, Tapped Delay/1
  Gain3/1 -> Sum15/1, Tapped Delay3/1
  Gain1/1 -> Sum15/3, Tapped Delay1/1
  Gain2/1 -> Sum15/2, Tapped Delay2/1
  Tapped Delay2/1 -> Sum of Elements2/1
  Gain5/1 -> [vxwOpt_FR]
  Gain6/1 -> [vxwOpt_RL]
  Tapped Delay3/1 -> Sum of Elements3/1
  Sum15/1 -> Gain13/1
  Gain13/1 -> [vxwMeanIn]
  Gain7/1 -> [vxwOpt_RR]
  Tapped Delay1/1 -> Sum of Elements1/1
  Tapped Delay/1 -> Sum of Elements/1
  FLwheelspeed_kmh/1 -> Product1/1
  FRwheelspeed_kmh/1 -> Product2/1
  RRwheelspeed_kmh/1 -> Product4/1
  RLwheelspeed_kmh/1 -> Product3/1

== system PvtSubSys_VIE/VIE/VIE/AxRef/LP filter ==
  Raw : Inport
  FilterTime : Constant  Value=0.05
  Memory2 : Memory  InheritSampleTime=on
  Product1 : Product  RndMeth=Zero
  Product4 : Product  Inputs=*/  RndMeth=Zero
  Sum4 : Sum  Inputs=+-|
  Sum5 : Sum  Inputs=++|
  Weight/N3 : Constant  Value=0.02
  output : Outport
  wires:
  Memory2/1 -> Sum4/2, Sum5/2
  Sum4/1 -> Product1/2
  Sum5/1 -> Memory2/1, output/1
  Product1/1 -> Sum5/1
  Raw/1 -> Sum4/1
  Weight/N3/1 -> Product4/1
  Product4/1 -> Product1/1
  FilterTime/1 -> Product4/2

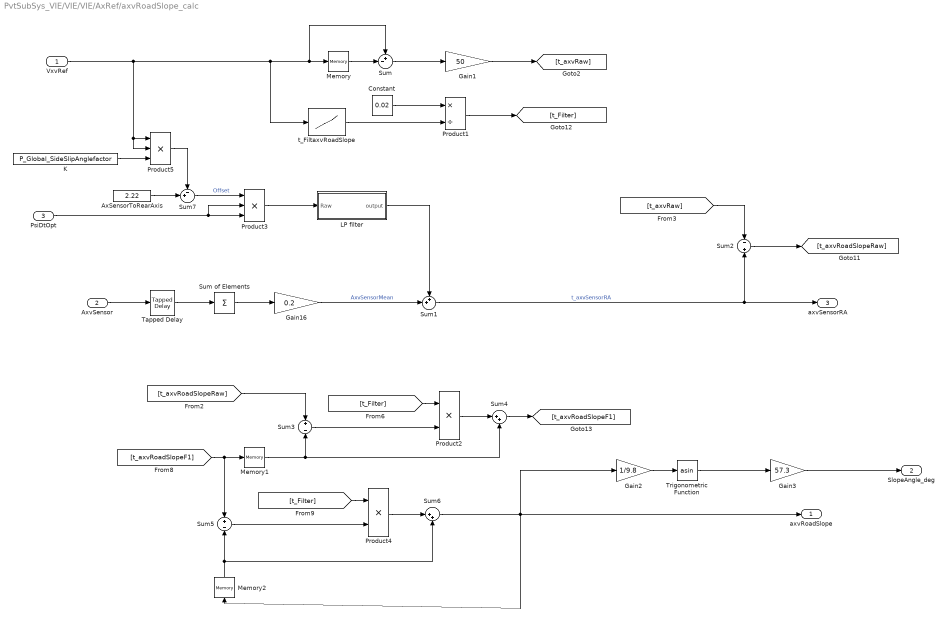
== system PvtSubSys_VIE/VIE/VIE/AxRef/axvRoadSlope_calc ==
  VxvRef : Inport
  AxvSensor : Inport  Port=2
  PsiDtOpt : Inport  Port=3
  AxSensorToRearAxis : Constant  Value=2.22  OutDataTypeStr=single
  Constant : Constant  Value=0.02  OutDataTypeStr=single
  Gain1 : Gain  Gain=50
  Gain16 : Gain  Gain=0.2
  Gain2 : Gain  Gain=1/9.8
  Gain3 : Gain  Gain=57.3
  K : Constant  Value=P_Global_SideSlipAnglefactor
  LP filter : Subsystem
  Memory : Memory  InheritSampleTime=on
  Memory1 : Memory  InheritSampleTime=on
  Memory2 : Memory  InheritSampleTime=on
  Product1 : Product  Inputs=*/  RndMeth=Zero
  Product2 : Product  RndMeth=Zero
  Product3 : Product  Inputs=3  RndMeth=Zero
  Product4 : Product  RndMeth=Zero
  Product5 : Product  Inputs=3  RndMeth=Zero
  Sum : Sum  Inputs=+-|
  Sum of Elements : Sum  Inputs=+
  Sum1 : Sum  Inputs=++|
  Sum2 : Sum  Inputs=-+
  Sum3 : Sum  Inputs=+-
  Sum4 : Sum  Inputs=|++
  Sum5 : Sum  Inputs=+-
  Sum6 : Sum  Inputs=|++
  Sum7 : Sum  Inputs=-+|
  Tapped Delay : simulink/Discrete/Tapped Delay  vinit=0.0  samptime=-1  NumDelays=4  DelayOrder=Newest  includeCurrent=on
  Trigonometric Function : Trigonometry  Operator=asin
  t_FiltaxvRoadSlope : Lookup_n-D  NumberOfTableDimensions=1  BreakpointsForDimension1=[0,41.7,55.6,80]  Table=[0.5,0.5,0.9,0.9]  RndMeth=Simplest  InputSameDT=on
  axvRoadSlope : Outport
  SlopeAngle_deg : Outport  Port=2
  axvSensorRA : Outport  Port=3
  wires:
  PsiDtOpt/1 -> Product3/3, Product3/2
  LP filter/1(output) -> Sum1/1
  K/1 -> Product5/3
  Product5/1 -> Sum7/1
  Sum7/1 -> Product3/1  "Offset"
  AxSensorToRearAxis/1 -> Sum7/2
  Gain3/1 -> SlopeAngle_deg/1
  Trigonometric Function/1 -> Gain3/1
  Gain2/1 -> Trigonometric Function/1
  [t_axvRaw] -> Sum2/1
  Product4/1 -> Sum6/1
  Sum5/1 -> Product4/2
  Product2/1 -> Sum4/1
  Sum6/1 -> axvRoadSlope/1, Gain2/1, Memory2/1
  [t_Filter] -> Product4/1
  Sum3/1 -> Product2/2
  [t_Filter] -> Product2/1
  [t_axvRoadSlopeF1] -> Memory1/1, Sum5/1
  Constant/1 -> Product1/1
  Memory1/1 -> Sum4/2, Sum3/2
  Memory2/1 -> Sum5/2, Sum6/2
  [t_axvRoadSlopeRaw] -> Sum3/1
  Sum4/1 -> [t_axvRoadSlopeF1]
  Product1/1 -> [t_Filter]
  t_FiltaxvRoadSlope/1 -> Product1/2
  VxvRef/1 -> Memory/1, Sum/1, t_FiltaxvRoadSlope/1, Product5/1, Product5/2
  Sum1/1 -> Sum2/2, axvSensorRA/1  "t_axvSensorRA"
  Sum2/1 -> [t_axvRoadSlopeRaw]
  Product3/1 -> LP filter/1(Raw)
  Gain1/1 -> [t_axvRaw]
  Sum/1 -> Gain1/1
  Gain16/1 -> Sum1/2  "AxvSensorMean"
  Sum of Elements/1 -> Gain16/1
  Tapped Delay/1 -> Sum of Elements/1
  AxvSensor/1 -> Tapped Delay/1
  Memory/1 -> Sum/2

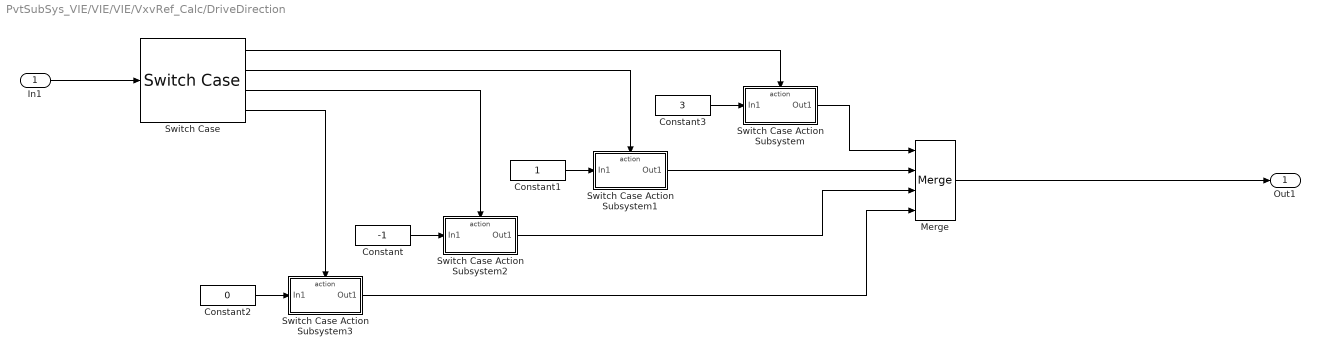
== system PvtSubSys_VIE/VIE/VIE/VxvRef_Calc/DriveDirection ==
  In1 : Inport
  Constant : Constant  Value=-1  OutDataTypeStr=single
  Constant1 : Constant  OutDataTypeStr=single
  Constant2 : Constant  Value=0  OutDataTypeStr=single
  Constant3 : Constant  Value=3  OutDataTypeStr=single
  Merge : Merge  Inputs=4
  Switch Case : SwitchCase  CaseConditions={0,1,2}
  Switch Case Action Subsystem : Subsystem  TreatAsAtomicUnit=on
  Switch Case Action Subsystem1 : Subsystem  TreatAsAtomicUnit=on
  Switch Case Action Subsystem2 : Subsystem  TreatAsAtomicUnit=on
  Switch Case Action Subsystem3 : Subsystem  TreatAsAtomicUnit=on
  Out1 : Outport
  wires:
  Constant/1 -> Switch Case Action Subsystem2/1(In1)
  Merge/1 -> Out1/1
  Constant1/1 -> Switch Case Action Subsystem1/1(In1)
  Switch Case Action Subsystem2/1(Out1) -> Merge/3
  Constant2/1 -> Switch Case Action Subsystem3/1(In1)
  Switch Case Action Subsystem3/1(Out1) -> Merge/4
  Switch Case/2 -> Switch Case Action Subsystem1/Action
  Switch Case Action Subsystem/1(Out1) -> Merge/1
  Switch Case/1 -> Switch Case Action Subsystem/Action
  Switch Case Action Subsystem1/1(Out1) -> Merge/2
  Constant3/1 -> Switch Case Action Subsystem/1(In1)
  Switch Case/4 -> Switch Case Action Subsystem3/Action
  Switch Case/3 -> Switch Case Action Subsystem2/Action
  In1/1 -> Switch Case/1

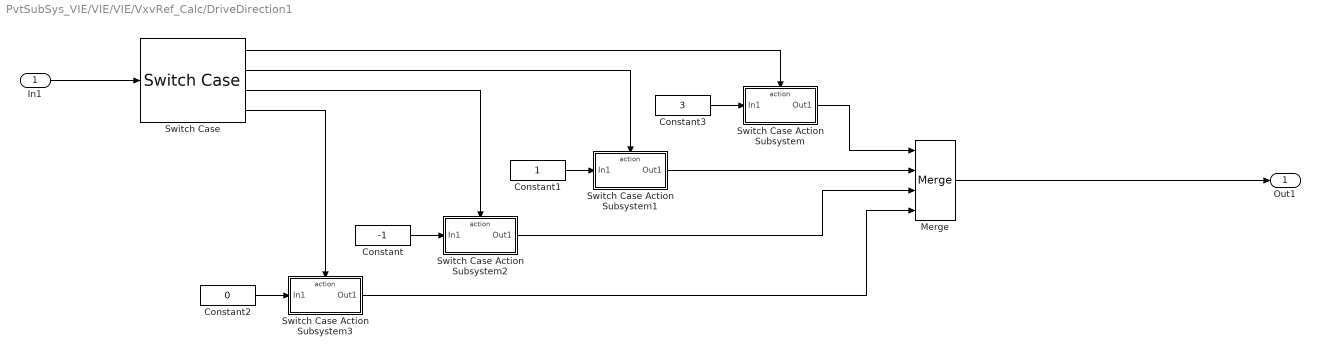
== system PvtSubSys_VIE/VIE/VIE/VxvRef_Calc/DriveDirection1 ==
  In1 : Inport
  Constant : Constant  Value=-1  OutDataTypeStr=single
  Constant1 : Constant  OutDataTypeStr=single
  Constant2 : Constant  Value=0  OutDataTypeStr=single
  Constant3 : Constant  Value=3  OutDataTypeStr=single
  Merge : Merge  Inputs=4
  Switch Case : SwitchCase  CaseConditions={0,1,2}
  Switch Case Action Subsystem : Subsystem  TreatAsAtomicUnit=on
  Switch Case Action Subsystem1 : Subsystem  TreatAsAtomicUnit=on
  Switch Case Action Subsystem2 : Subsystem  TreatAsAtomicUnit=on
  Switch Case Action Subsystem3 : Subsystem  TreatAsAtomicUnit=on
  Out1 : Outport
  wires:
  Constant/1 -> Switch Case Action Subsystem2/1(In1)
  Merge/1 -> Out1/1
  Constant1/1 -> Switch Case Action Subsystem1/1(In1)
  Switch Case Action Subsystem2/1(Out1) -> Merge/3
  Constant2/1 -> Switch Case Action Subsystem3/1(In1)
  Switch Case Action Subsystem3/1(Out1) -> Merge/4
  Switch Case/2 -> Switch Case Action Subsystem1/Action
  Switch Case Action Subsystem/1(Out1) -> Merge/1
  Switch Case/1 -> Switch Case Action Subsystem/Action
  Switch Case Action Subsystem1/1(Out1) -> Merge/2
  Constant3/1 -> Switch Case Action Subsystem/1(In1)
  Switch Case/4 -> Switch Case Action Subsystem3/Action
  Switch Case/3 -> Switch Case Action Subsystem2/Action
  In1/1 -> Switch Case/1

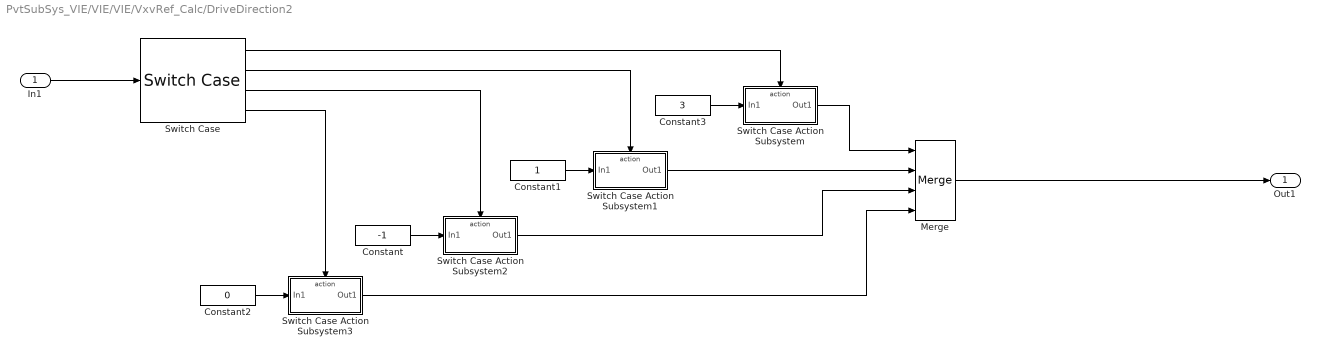
== system PvtSubSys_VIE/VIE/VIE/VxvRef_Calc/DriveDirection2 ==
  In1 : Inport
  Constant : Constant  Value=-1  OutDataTypeStr=single
  Constant1 : Constant  OutDataTypeStr=single
  Constant2 : Constant  Value=0  OutDataTypeStr=single
  Constant3 : Constant  Value=3  OutDataTypeStr=single
  Merge : Merge  Inputs=4
  Switch Case : SwitchCase  CaseConditions={0,1,2}
  Switch Case Action Subsystem : Subsystem  TreatAsAtomicUnit=on
  Switch Case Action Subsystem1 : Subsystem  TreatAsAtomicUnit=on
  Switch Case Action Subsystem2 : Subsystem  TreatAsAtomicUnit=on
  Switch Case Action Subsystem3 : Subsystem  TreatAsAtomicUnit=on
  Out1 : Outport
  wires:
  Constant/1 -> Switch Case Action Subsystem2/1(In1)
  Merge/1 -> Out1/1
  Constant1/1 -> Switch Case Action Subsystem1/1(In1)
  Switch Case Action Subsystem2/1(Out1) -> Merge/3
  Constant2/1 -> Switch Case Action Subsystem3/1(In1)
  Switch Case Action Subsystem3/1(Out1) -> Merge/4
  Switch Case/2 -> Switch Case Action Subsystem1/Action
  Switch Case Action Subsystem/1(Out1) -> Merge/1
  Switch Case/1 -> Switch Case Action Subsystem/Action
  Switch Case Action Subsystem1/1(Out1) -> Merge/2
  Constant3/1 -> Switch Case Action Subsystem/1(In1)
  Switch Case/4 -> Switch Case Action Subsystem3/Action
  Switch Case/3 -> Switch Case Action Subsystem2/Action
  In1/1 -> Switch Case/1

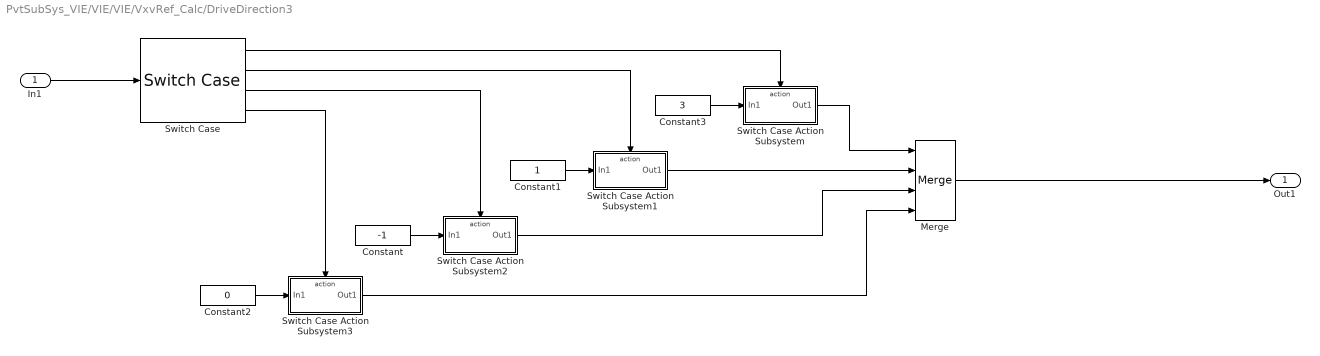
== system PvtSubSys_VIE/VIE/VIE/VxvRef_Calc/DriveDirection3 ==
  In1 : Inport
  Constant : Constant  Value=-1  OutDataTypeStr=single
  Constant1 : Constant  OutDataTypeStr=single
  Constant2 : Constant  Value=0  OutDataTypeStr=single
  Constant3 : Constant  Value=3  OutDataTypeStr=single
  Merge : Merge  Inputs=4
  Switch Case : SwitchCase  CaseConditions={0,1,2}
  Switch Case Action Subsystem : Subsystem  TreatAsAtomicUnit=on
  Switch Case Action Subsystem1 : Subsystem  TreatAsAtomicUnit=on
  Switch Case Action Subsystem2 : Subsystem  TreatAsAtomicUnit=on
  Switch Case Action Subsystem3 : Subsystem  TreatAsAtomicUnit=on
  Out1 : Outport
  wires:
  Constant/1 -> Switch Case Action Subsystem2/1(In1)
  Merge/1 -> Out1/1
  Constant1/1 -> Switch Case Action Subsystem1/1(In1)
  Switch Case Action Subsystem2/1(Out1) -> Merge/3
  Constant2/1 -> Switch Case Action Subsystem3/1(In1)
  Switch Case Action Subsystem3/1(Out1) -> Merge/4
  Switch Case/2 -> Switch Case Action Subsystem1/Action
  Switch Case Action Subsystem/1(Out1) -> Merge/1
  Switch Case/1 -> Switch Case Action Subsystem/Action
  Switch Case Action Subsystem1/1(Out1) -> Merge/2
  Constant3/1 -> Switch Case Action Subsystem/1(In1)
  Switch Case/4 -> Switch Case Action Subsystem3/Action
  Switch Case/3 -> Switch Case Action Subsystem2/Action
  In1/1 -> Switch Case/1

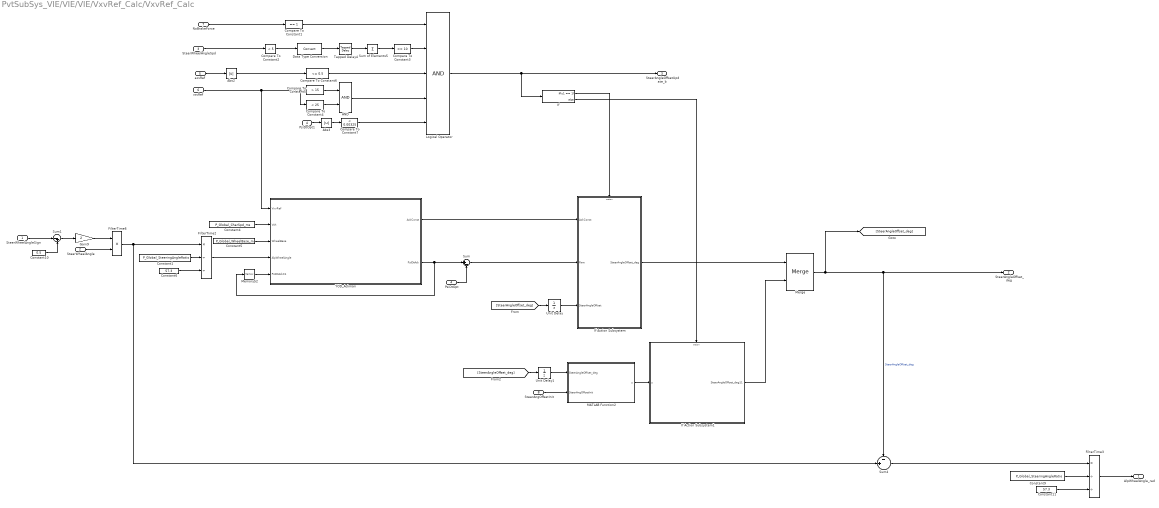
== system PvtSubSys_VIE/VIE/VIE/VxvRef_Calc/VxvRef_Calc ==
  SteerWheelAngleSign : Inport
  SteerWheelAngle : Inport  Port=2
  SteerWheelAngleSpd : Inport  Port=3
  PsiDtOpt : Inport  Port=4
  axvRef : Inport  Port=5
  vxvRef : Inport  Port=6
  NoBrakeForce : Inport  Port=7
  SteerAngOffsetInit : Inport  Port=8
  AND : Logic  AllPortsSameDT=off  OutDataTypeStr=boolean
  Abs2 : Abs
  Abs3 : Abs
  Compare To Constant1 : simulink/Logic and Bit Operations/Compare To Constant  relop===  const=1  OutDataTypeStr=boolean
  Compare To Constant2 : simulink/Logic and Bit Operations/Compare To Constant  relop=<  const=5  OutDataTypeStr=boolean
  Compare To Constant3 : simulink/Logic and Bit Operations/Compare To Constant  relop===  const=10  OutDataTypeStr=boolean
  Compare To Constant4 : simulink/Logic and Bit Operations/Compare To Constant  relop=<  const=25  OutDataTypeStr=boolean
  Compare To Constant5 : simulink/Logic and Bit Operations/Compare To Constant  relop=>  const=15  OutDataTypeStr=boolean
  Compare To Constant6 : simulink/Logic and Bit Operations/Compare To Constant  relop=<=  const=0.5  OutDataTypeStr=boolean
  Compare To Constant7 : simulink/Logic and Bit Operations/Compare To Constant  relop=<  const=0.00325  OutDataTypeStr=boolean
  Constant1 : Constant  Value=P_Global_SteeringAngleRatio
  Constant10 : Constant  Value=0.5  OutDataTypeStr=single
  Constant11 : Constant  Value=57.3  OutDataTypeStr=single
  Constant4 : Constant  Value=P_Global_CharSpd_ms
  Constant5 : Constant  Value=P_Global_WheelBase_m
  Constant6 : Constant  Value=57.3  OutDataTypeStr=single
  Constant9 : Constant  Value=P_Global_SteeringAngleRatio
  Data Type Conversion : DataTypeConversion
  FilterTime2 : Product  Inputs=*//  RndMeth=Zero
  FilterTime3 : Product  Inputs=*//  RndMeth=Zero
  FilterTime6 : Product  Inputs=**  RndMeth=Zero
  Gain9 : Gain  Gain=2
  If : If  IfExpression=u1 == 1
  If Action Subsystem : Subsystem  TreatAsAtomicUnit=on
  If Action Subsystem1 : Subsystem  TreatAsAtomicUnit=on
  Logical Operator : Logic  Inputs=5  AllPortsSameDT=off  OutDataTypeStr=boolean
  MATLAB Function2 : MATLAB Function  TreatAsAtomicUnit=on
  Memory52 : Memory  InheritSampleTime=on
  Merge : Merge
  PsiDtOpt1 : InportShadow  Port=4
  Sum : Sum  Inputs=|+-
  Sum of Elements5 : Sum  Inputs=+
  Sum1 : Sum  Inputs=|-+
  Sum4 : Sum  Inputs=-+|
  Tapped Delay4 : simulink/Discrete/Tapped Delay  vinit=0.0  samptime=-1  NumDelays=9  DelayOrder=Newest  includeCurrent=on
  Unit Delay : UnitDelay  SampleTime=-1  HasFrameUpgradeWarning=on
  Unit Delay1 : UnitDelay  SampleTime=-1  HasFrameUpgradeWarning=on
  YOD_Ackman : MATLAB Function  TreatAsAtomicUnit=on
  AlpWheelAngle_rad : Outport
  SteerAngleOffset_deg : Outport  Port=2
  SteerAngleOffsetUpdate_b : Outport  Port=3
  wires:
  MATLAB Function2/1(y) -> If Action Subsystem1/1(y)
  SteerAngOffsetInit/1 -> MATLAB Function2/2(SteerAngOffsetInit)
  Unit Delay1/1 -> MATLAB Function2/1(SteerAngleOffset_deg)
  If/2 -> If Action Subsystem1/Action
  If Action Subsystem1/1(SteerAngleOffset_deg11) -> Merge/2
  If Action Subsystem/1(SteerAngleOffset_deg) -> Merge/1
  If/1 -> If Action Subsystem/Action
  [SteerAngleOffset_deg] -> Unit Delay1/1
  Unit Delay/1 -> If Action Subsystem/3(SteerAngleOffset)
  [SteerAngleOffset_deg] -> Unit Delay/1
  Compare To Constant4/1 -> AND/2
  Compare To Constant5/1 -> AND/1
  Compare To Constant7/1 -> Logical Operator/5
  Abs3/1 -> Compare To Constant7/1
  PsiDtOpt1/1 -> Abs3/1
  Compare To Constant1/1 -> Logical Operator/1
  NoBrakeForce/1 -> Compare To Constant1/1
  Compare To Constant6/1 -> Logical Operator/3
  Abs2/1 -> Compare To Constant6/1
  axvRef/1 -> Abs2/1
  FilterTime3/1 -> AlpWheelAngle_rad/1
  Sum4/1 -> FilterTime3/1
  Constant11/1 -> FilterTime3/3
  Constant9/1 -> FilterTime3/2
  FilterTime2/1 -> YOD_Ackman/4(AlpWheelAngle)
  Merge/1 -> [SteerAngleOffset_deg], Sum4/1, SteerAngleOffset_deg/1  "SteerAngleOffset_deg"
  YOD_Ackman/1(AckConst) -> If Action Subsystem/1(AckConst)
  Constant6/1 -> FilterTime2/3
  Constant1/1 -> FilterTime2/2
  FilterTime6/1 -> Sum4/2, FilterTime2/1
  Logical Operator/1 -> If/1, SteerAngleOffsetUpdate_b/1
  Sum/1 -> If Action Subsystem/2(Raw)
  AND/1 -> Logical Operator/4
  vxvRef/1 -> Compare To Constant5/1, Compare To Constant4/1, YOD_Ackman/1(VxvRef)
  Compare To Constant3/1 -> Logical Operator/2
  PsiDtOpt/1 -> Sum/2
  Data Type Conversion/1 -> Tapped Delay4/1
  Compare To Constant2/1 -> Data Type Conversion/1
  Sum of Elements5/1 -> Compare To Constant3/1
  Tapped Delay4/1 -> Sum of Elements5/1
  SteerWheelAngleSpd/1 -> Compare To Constant2/1
  Sum1/1 -> Gain9/1
  SteerWheelAngle/1 -> FilterTime6/2
  Gain9/1 -> FilterTime6/1
  SteerWheelAngleSign/1 -> Sum1/1
  Constant10/1 -> Sum1/2
  Memory52/1 -> YOD_Ackman/5(PsiDtAckK1)
  Constant4/1 -> YOD_Ackman/2(Vch)
  YOD_Ackman/2(PsiDtAck) -> Memory52/1, Sum/1
  Constant5/1 -> YOD_Ackman/3(WheelBase)

== system PvtSubSys_VIE/VIE/VIE/AxRef/axvRoadSlope_calc/LP filter ==
  Raw : Inport
  FilterTime : Constant  Value=0.05  OutDataTypeStr=single
  Memory2 : Memory  InheritSampleTime=on
  Product1 : Product  RndMeth=Zero
  Product4 : Product  Inputs=*/  RndMeth=Zero
  Sum4 : Sum  Inputs=+-|
  Sum5 : Sum  Inputs=++|
  Weight/N3 : Constant  Value=0.02  OutDataTypeStr=single
  output : Outport
  wires:
  Memory2/1 -> Sum4/2, Sum5/2
  Sum4/1 -> Product1/2
  Sum5/1 -> Memory2/1, output/1
  Product1/1 -> Sum5/1
  Raw/1 -> Sum4/1
  Weight/N3/1 -> Product4/1
  Product4/1 -> Product1/1
  FilterTime/1 -> Product4/2

== system PvtSubSys_VIE/VIE/VIE/VxvRef_Calc/DriveDirection/Switch Case Action Subsystem ==
  In1 : Inport
  Action Port : ActionPort
  Out1 : Outport
  wires:
  In1/1 -> Out1/1

== system PvtSubSys_VIE/VIE/VIE/VxvRef_Calc/DriveDirection/Switch Case Action Subsystem1 ==
  In1 : Inport
  Action Port : ActionPort
  Out1 : Outport
  wires:
  In1/1 -> Out1/1

== system PvtSubSys_VIE/VIE/VIE/VxvRef_Calc/DriveDirection/Switch Case Action Subsystem2 ==
  In1 : Inport
  Action Port : ActionPort
  Out1 : Outport
  wires:
  In1/1 -> Out1/1

== system PvtSubSys_VIE/VIE/VIE/VxvRef_Calc/DriveDirection/Switch Case Action Subsystem3 ==
  In1 : Inport
  Action Port : ActionPort
  Out1 : Outport
  wires:
  In1/1 -> Out1/1

== system PvtSubSys_VIE/VIE/VIE/VxvRef_Calc/DriveDirection1/Switch Case Action Subsystem ==
  In1 : Inport
  Action Port : ActionPort
  Out1 : Outport
  wires:
  In1/1 -> Out1/1

== system PvtSubSys_VIE/VIE/VIE/VxvRef_Calc/DriveDirection1/Switch Case Action Subsystem1 ==
  In1 : Inport
  Action Port : ActionPort
  Out1 : Outport
  wires:
  In1/1 -> Out1/1

== system PvtSubSys_VIE/VIE/VIE/VxvRef_Calc/DriveDirection1/Switch Case Action Subsystem2 ==
  In1 : Inport
  Action Port : ActionPort
  Out1 : Outport
  wires:
  In1/1 -> Out1/1

== system PvtSubSys_VIE/VIE/VIE/VxvRef_Calc/DriveDirection1/Switch Case Action Subsystem3 ==
  In1 : Inport
  Action Port : ActionPort
  Out1 : Outport
  wires:
  In1/1 -> Out1/1

== system PvtSubSys_VIE/VIE/VIE/VxvRef_Calc/DriveDirection2/Switch Case Action Subsystem ==
  In1 : Inport
  Action Port : ActionPort
  Out1 : Outport
  wires:
  In1/1 -> Out1/1

== system PvtSubSys_VIE/VIE/VIE/VxvRef_Calc/DriveDirection2/Switch Case Action Subsystem1 ==
  In1 : Inport
  Action Port : ActionPort
  Out1 : Outport
  wires:
  In1/1 -> Out1/1

== system PvtSubSys_VIE/VIE/VIE/VxvRef_Calc/DriveDirection2/Switch Case Action Subsystem2 ==
  In1 : Inport
  Action Port : ActionPort
  Out1 : Outport
  wires:
  In1/1 -> Out1/1

== system PvtSubSys_VIE/VIE/VIE/VxvRef_Calc/DriveDirection2/Switch Case Action Subsystem3 ==
  In1 : Inport
  Action Port : ActionPort
  Out1 : Outport
  wires:
  In1/1 -> Out1/1

== system PvtSubSys_VIE/VIE/VIE/VxvRef_Calc/DriveDirection3/Switch Case Action Subsystem ==
  In1 : Inport
  Action Port : ActionPort
  Out1 : Outport
  wires:
  In1/1 -> Out1/1

== system PvtSubSys_VIE/VIE/VIE/VxvRef_Calc/DriveDirection3/Switch Case Action Subsystem1 ==
  In1 : Inport
  Action Port : ActionPort
  Out1 : Outport
  wires:
  In1/1 -> Out1/1

== system PvtSubSys_VIE/VIE/VIE/VxvRef_Calc/DriveDirection3/Switch Case Action Subsystem2 ==
  In1 : Inport
  Action Port : ActionPort
  Out1 : Outport
  wires:
  In1/1 -> Out1/1

== system PvtSubSys_VIE/VIE/VIE/VxvRef_Calc/DriveDirection3/Switch Case Action Subsystem3 ==
  In1 : Inport
  Action Port : ActionPort
  Out1 : Outport
  wires:
  In1/1 -> Out1/1

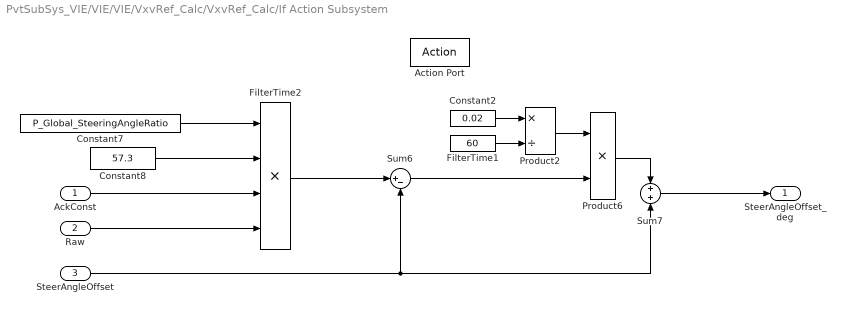
== system PvtSubSys_VIE/VIE/VIE/VxvRef_Calc/VxvRef_Calc/If Action Subsystem ==
  AckConst : Inport
  Raw : Inport  Port=2
  SteerAngleOffset : Inport  Port=3
  Action Port : ActionPort
  Constant2 : Constant  Value=0.02  OutDataTypeStr=single
  Constant7 : Constant  Value=P_Global_SteeringAngleRatio
  Constant8 : Constant  Value=57.3  OutDataTypeStr=single
  FilterTime1 : Constant  Value=60  OutDataTypeStr=single
  FilterTime2 : Product  Inputs=4  RndMeth=Zero
  Product2 : Product  Inputs=*/  RndMeth=Zero
  Product6 : Product  RndMeth=Zero
  Sum6 : Sum  Inputs=|+-
  Sum7 : Sum
  SteerAngleOffset_deg : Outport
  wires:
  Constant8/1 -> FilterTime2/2
  Constant2/1 -> Product2/1
  Sum7/1 -> SteerAngleOffset_deg/1
  Product6/1 -> Sum7/1
  Product2/1 -> Product6/1
  FilterTime1/1 -> Product2/2
  Constant7/1 -> FilterTime2/1
  Sum6/1 -> Product6/2
  Raw/1 -> FilterTime2/4
  FilterTime2/1 -> Sum6/1
  AckConst/1 -> FilterTime2/3
  SteerAngleOffset/1 -> Sum6/2, Sum7/2

== system PvtSubSys_VIE/VIE/VIE/VxvRef_Calc/VxvRef_Calc/If Action Subsystem1 ==
  y : Inport
  Action Port : ActionPort
  SteerAngleOffset_deg11 : Outport
  wires:
  y/1 -> SteerAngleOffset_deg11/1

== matlab function PvtSubSys_VIE/VIE/VIE/VxvRef_Calc/calcVxwDiffAndModErr_v ==
  data: t_vxwCorrFL input; t_vxwCorrMax output; t_vxwCorrFR input; t_vxwCorrRL input; t_vxwCorrMin output; ErrWheel_FL output; ErrWheel_FR output; t_vxwCorrRR input; ErrWheel_RL output; ErrWheel_RR output
function [t_vxwCorrMax,t_vxwCorrMin,ErrWheel_FL,ErrWheel_FR,ErrWheel_RL,ErrWheel_RR] = fcn(t_vxwCorrFL,t_vxwCorrFR,t_vxwCorrRL,t_vxwCorrRR)
%#codegen
t_temp1 = min(t_vxwCorrFL,t_vxwCorrFR);
t_temp1 = min(t_temp1,t_vxwCorrRL);
t_vxwCorrMin = min(t_temp1,t_vxwCorrRR);

t_temp1 = max(t_vxwCorrFL,t_vxwCorrFR);
t_temp1 = max(t_temp1,t_vxwCorrRL);
t_vxwCorrMax = max(t_temp1,t_vxwCorrRR);

t_vxwDiffMax = t_vxwCorrMax - t_vxwCorrMin;

 t_vxwDiffFLFR =abs(t_vxwCorrFL - t_vxwCorrFR);  
 t_vxwDiffFLRL =abs(t_vxwCorrFL - t_vxwCorrRL); 
 t_vxwDiffFLRR =abs(t_vxwCorrFL - t_vxwCorrRR); 
 t_vxwDiffFRRL =abs(t_vxwCorrFR - t_vxwCorrRL);  
 t_vxwDiffFRRR =abs(t_vxwCorrFR - t_vxwCorrRR); 
 t_vxwDiffRLRR =abs(t_vxwCorrRL - t_vxwCorrRR);
 
 t_vxwDiffAllowed = single(0.6)*t_vxwDiffMax;% 常数值转为single型
 
 if (t_vxwDiffFLFR>t_vxwDiffAllowed)&&(t_vxwDiffFLRL>t_vxwDiffAllowed)&&(t_vxwDiffFLRR>t_vxwDiffAllowed)
     ErrWheel_FL = uint8(1);% 常数值转为single型
 else
     ErrWheel_FL = uint8(0);% 常数值转为uint8型
 end
 if (t_vxwDiffFLFR>t_vxwDiffAllowed)&&(t_vxwDiffFRRL>t_vxwDiffAllowed)&&(t_vxwDiffFRRR>t_vxwDiffAllowed)
     ErrWheel_FR = uint8(1);% 常数值转为uint8型
 else
     ErrWheel_FR = uint8(0);% 常数值转为uint8型
 end
 if (t_vxwDiffFLRL>t_vxwDiffAllowed)&&(t_vxwDiffFRRL>t_vxwDiffAllowed)&&(t_vxwDiffRLRR>t_vxwDiffAllowed)
     ErrWheel_RL = uint8(1);% 常数值转为uint8型
 else
     ErrWheel_RL = uint8(0);% 常数值转为uint8型
 end
 if (t_vxwDiffFLRR>t_vxwDiffAllowed)&&(t_vxwDiffFRRR>t_vxwDiffAllowed)&&(t_vxwDiffRLRR>t_vxwDiffAllowed)
     ErrWheel_RR = uint8(1);% 常数值转为uint8型
 else
     ErrWheel_RR = uint8(0);% 常数值转为uint8型
 end

== matlab function PvtSubSys_VIE/VIE/VIE/VxvRef_Calc/detErrorBandMax ==
  data: t_vxwCorrFL input; l_vxwMax_aswFL output; t_vxwCorrFR input; t_vxwCorrRL input; t_vxwCorrRR input; l_vxwMax_aswFR output; ErrWheel_FL input; ErrWheel_FR input; ErrWheel_RL input; ErrWheel_RR input; t_SlipBrake input; l_CaseBrake input; l_vxwMax_aswRL output; l_vxwMax_aswRR output
function [l_vxwMax_aswFL,l_vxwMax_aswFR,l_vxwMax_aswRL,l_vxwMax_aswRR] = fcn(t_vxwCorrFL,t_vxwCorrFR,t_vxwCorrRL,t_vxwCorrRR,ErrWheel_FL,ErrWheel_FR,ErrWheel_RL,ErrWheel_RR,t_SlipBrake,l_CaseBrake)
%#codegen
t_vxwErrBandMax=single(-128);%转换常数数据类型
if ErrWheel_FL==uint8(0)%转换常数数据类型
    t_vxwMax = t_vxwCorrFL*(single(1) + t_SlipBrake);%转换常数数据类型
    t_vxwErrBandMax = max(t_vxwErrBandMax,t_vxwMax);
    l_vxwMax_aswFL = t_vxwMax;
else
    l_vxwMax_aswFL = single(128);%转换常数数据类型
end

if ErrWheel_FR==uint8(0)%转换常数数据类型
    t_vxwMax = t_vxwCorrFR*(single(1) + t_SlipBrake);%转换常数数据类型
    t_vxwErrBandMax = max(t_vxwErrBandMax,t_vxwMax);
    l_vxwMax_aswFR = t_vxwMax;
else
    l_vxwMax_aswFR = single(128);%转换常数数据类型
end

if ErrWheel_RL==uint8(0)%转换常数数据类型
    t_vxwMax = t_vxwCorrRL*(single(1) + t_SlipBrake);%转换常数数据类型
    t_vxwErrBandMax = max(t_vxwErrBandMax,t_vxwMax);
    l_vxwMax_aswRL = t_vxwMax;
else
    l_vxwMax_aswRL = single(128);%转换常数数据类型
end

if ErrWheel_RR==uint8(0)%转换常数数据类型
    t_vxwMax = t_vxwCorrRR*(single(1) + t_SlipBrake);%转换常数数据类型
    t_vxwErrBandMax = max(t_vxwErrBandMax,t_vxwMax);
    l_vxwMax_aswRR = t_vxwMax;
else
    l_vxwMax_aswRR = single(128);%转换常数数据类型
end

if l_CaseBrake==uint8(1)%转换常数数据类型
    l_vxwMax_aswFL = t_vxwErrBandMax;
    l_vxwMax_aswFR = t_vxwErrBandMax;
    l_vxwMax_aswRL = t_vxwErrBandMax;
    l_vxwMax_aswRR = t_vxwErrBandMax;
end

== matlab function PvtSubSys_VIE/VIE/VIE/VxvRef_Calc/detErrorBandMin ==
  data: t_vxwCorrFL input; t_vxwCorrFR input; t_vxwCorrRL input; t_vxwCorrRR input; l_vxwMin_aswFR output size=1; ErrWheel_FL input; ErrWheel_FR input; ErrWheel_RL input; ErrWheel_RR input; t_SlipDrive input; l_CaseBrake input; l_vxwMin_aswRL output size=1; l_vxwMin_aswRR output size=1; FrontDrive input; RearDrive input; l_vxwMin_aswFL output size=1
function [l_vxwMin_aswFR,l_vxwMin_aswRL,l_vxwMin_aswRR, l_vxwMin_aswFL] = fcn(t_vxwCorrFL,t_vxwCorrFR,t_vxwCorrRL,t_vxwCorrRR,ErrWheel_FL,ErrWheel_FR,ErrWheel_RL,ErrWheel_RR,t_SlipDrive,l_CaseBrake,FrontDrive,RearDrive)
%#codegen
t_vxwErrBandMin = single(128);%转换常数数据类型
if ErrWheel_FL==uint8(0)%转换常数数据类型
    t_vxwMin = t_vxwCorrFL*(single(1) + single(FrontDrive)*single(t_SlipDrive));%转换常数及变量数据类型
    t_vxwErrBandMin = min(t_vxwErrBandMin,t_vxwMin);
    l_vxwMin_aswFL = t_vxwMin;
else
    l_vxwMin_aswFL = single(-128);%转换常数数据类型
end

if ErrWheel_FR==uint8(0)%转换常数数据类型
    t_vxwMin = t_vxwCorrFR*(single(1) + single(FrontDrive)*single(t_SlipDrive));%转换常数变量数据类型
    t_vxwErrBandMin = min(t_vxwErrBandMin,t_vxwMin);
    l_vxwMin_aswFR = t_vxwMin;
else
    l_vxwMin_aswFR = single(-128);%转换常数数据类型
end

if ErrWheel_RL==uint8(0)%转换常数数据类型
    t_vxwMin = t_vxwCorrRL*(single(1) + single(RearDrive)*single(t_SlipDrive));%转换常数变量数据类型
    t_vxwErrBandMin = min(t_vxwErrBandMin,t_vxwMin);
    l_vxwMin_aswRL = t_vxwMin;
else
    l_vxwMin_aswRL = single(-128);%转换常数数据类型
end

if ErrWheel_RR==uint8(0)%转换常数数据类型
    t_vxwMin = t_vxwCorrRR*(single(1) + single(RearDrive)*single(t_SlipDrive));%转换常数变量数据类型
    t_vxwErrBandMin = min(t_vxwErrBandMin,t_vxwMin);
    l_vxwMin_aswRR = t_vxwMin;
else
    l_vxwMin_aswRR = single(-128);%转换常数数据类型
end

if l_CaseBrake==uint8(0)%转换常数数据类型
    if FrontDrive==uint8(1)%转换常数数据类型
      l_vxwMin_aswFL = t_vxwErrBandMin;
      l_vxwMin_aswFR = t_vxwErrBandMin;
    end
    if RearDrive==uint8(1)%转换常数数据类型
      l_vxwMin_aswRL = t_vxwErrBandMin;
      l_vxwMin_aswRR = t_vxwErrBandMin;
    end
end
